simulink model "ModifiedBatteryModel3"  (R2019a)
settings: Solver=VariableStepAuto  StartTime=0.0  StopTime=10.0  RelTol=1e-3
libraries: fl_lib x6, nesl_utility x5
settings Model: Creator=nikos  LastModifiedBy=nikos

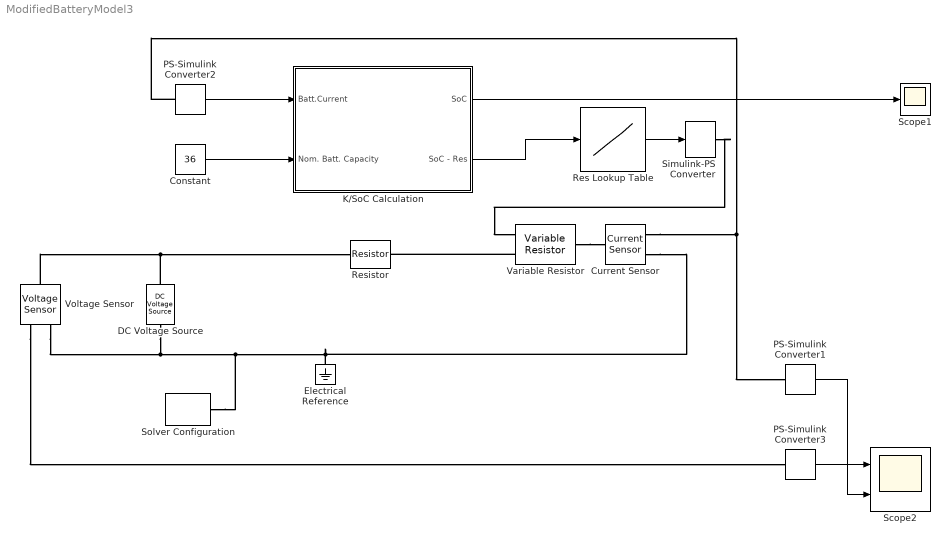
== system ModifiedBatteryModel3 ==
  Constant : Constant  Value=36
  Current Sensor : fl_lib/Electrical/Electrical Sensors/Current Sensor
  DC Voltage Source : fl_lib/Electrical/Electrical Sources/DC Voltage Source  v0=72 V
  Electrical Reference : fl_lib/Electrical/Electrical Elements/Electrical Reference
  K/SoC Calculation : Subsystem
  PS-Simulink Converter1 : nesl_utility/PS-Simulink Converter  PhysicalDomain=network_engine_domain  SubClassName=ps_output  LeftPortType=input  RightPortType=output  PseudoPeriodic=off  Frequencies=[]  Unit=1  AffineConversion=off
  PS-Simulink Converter2 : nesl_utility/PS-Simulink Converter  PhysicalDomain=network_engine_domain  SubClassName=ps_output  LeftPortType=input  RightPortType=output  PseudoPeriodic=off  Frequencies=[]  Unit=1  AffineConversion=off
  PS-Simulink Converter3 : nesl_utility/PS-Simulink Converter  PhysicalDomain=network_engine_domain  SubClassName=ps_output  LeftPortType=input  RightPortType=output  PseudoPeriodic=off  Frequencies=[]  Unit=1  AffineConversion=off
  Res Lookup Table : Lookup_n-D  NumberOfTableDimensions=1  BreakpointsForDimension1=[0, 10, 20, 30, 40, 50, 60, 70, 80, 90, 100]  Table=[0.011448, 0.011038, 0.011281, 0.011236, 0.010959, 0.010714, 0.010698, 0.010712, 0.010917, 0.011304, 0.011603]  InternalRulePriority=Speed  RndMeth=Simplest  InputSameDT=on
  Resistor : fl_lib/Electrical/Electrical Elements/Resistor  R=1.5 Ohm  i_specify=off  i_priority=High  i=0 A  i_nominal_specify=off  i_nominal_unit=A  i_nominal_value=1  v_specify=off  v_priority=High  v=0 V  v_nominal_specify=off  v_nominal_unit=V  v_nominal_value=1
  Scope1 : Scope
  Scope2 : Scope  NumInputPorts=2
  Simulink-PS Converter : nesl_utility/Simulink-PS Converter  PhysicalDomain=network_engine_domain  SubClassName=ps_input  LeftPortType=input  RightPortType=output  PseudoPeriodic=off  Frequencies=[]  NoiseDistribution=none  NoiseParameters=[]  Unit=1  AffineConversion=off  FilteringAndDerivatives=zero  SimscapeFilterOrder=1  InputFilterTimeConstant=0.001  UdotUserProvided=1
  Solver Configuration : nesl_utility/Solver Configuration  PhysicalDomain=network_engine_domain  SubClassName=solver  LeftPortType=input  RightPortType=generic  Tones=[]  Harmonics=[]  SimulateNoise=off  Profile=off  UseLocalSampling=off  EnableSwitchedLinearOptims=on  FrequencyDomain=off  UseCCode=off  RelTol=0.001  AbsTol=1e-06  MinStep=1e-09  ToWorkspace=off  RevertToSquareIcSolve=off  NumHomotopyIterations=100  PhasorMode=off  PhasorModeNumHarmonics=1  DoDC=off  ResidualTolerance=1e-09  UseLocalSolver=off  LocalSolverChoice=NE_BACKWARD_EULER_ADVANCER  LocalSolverSampleTime=0.001  DoFixedCost=off  MaxNonlinIter=3  MaxModeIter=2  LinearAlgebra=auto  EquationFormulation=NE_TIME_EF  DelaysMemoryBudget=1024  AutomaticFiltering=on  FilteringTimeConstant=0.001  PartitionStorageMethod=AS_NEEDED  PartitionMemoryBudget=1024  PartitionMethod=ROBUST
  Variable Resistor : fl_lib/Electrical/Electrical Elements/Variable Resistor  Rmin=0 Ohm  i_specify=off  i_priority=High  i=0 A  i_nominal_specify=off  i_nominal_unit=A  i_nominal_value=1  v_specify=off  v_priority=High  v=0 V  v_nominal_specify=off  v_nominal_unit=V  v_nominal_value=1
  Voltage Sensor : fl_lib/Electrical/Electrical Sensors/Voltage Sensor
  wires:
  Res Lookup Table/1 -> Simulink-PS Converter/1
  PS-Simulink Converter1/1 -> Scope2/2
  PS-Simulink Converter3/1 -> Scope2/1
  PS-Simulink Converter2/1 -> K/SoC Calculation/1(Batt.Current)
  Constant/1 -> K/SoC Calculation/2(Nom. Batt. Capacity)
  K/SoC Calculation/1(SoC) -> Scope1/1
  K/SoC Calculation/2(SoC - Res) -> Res Lookup Table/1
  connections:
  DC Voltage Source/LConn1 -- Voltage Sensor/LConn1 -- Resistor/LConn1
  DC Voltage Source/RConn1 -- Current Sensor/RConn2 -- Electrical Reference/LConn1 -- Solver Configuration/RConn1 -- Voltage Sensor/RConn2
  Variable Resistor/RConn1 -- Current Sensor/LConn1
  Simulink-PS Converter/RConn1 -- Variable Resistor/LConn1
  Variable Resistor/LConn2 -- Resistor/RConn1
  Voltage Sensor/RConn1 -- PS-Simulink Converter3/LConn1
  Current Sensor/RConn1 -- PS-Simulink Converter1/LConn1 -- PS-Simulink Converter2/LConn1

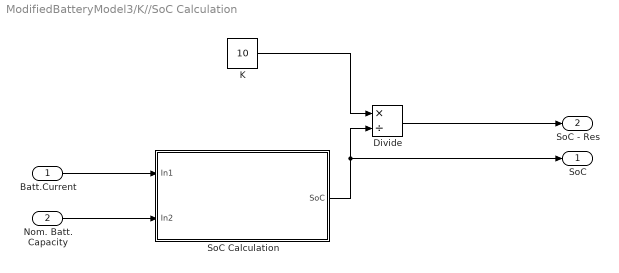
== system ModifiedBatteryModel3/K//SoC Calculation ==
  Batt.Current : Inport
  Nom. Batt. Capacity : Inport  Port=2
  Divide : Product  Inputs=*/
  K : Constant  Value=10
  SoC Calculation : Subsystem
  SoC : Outport
  SoC - Res : Outport  Port=2
  wires:
  SoC Calculation/1(" SoC") -> SoC/1, Divide/2
  Nom. Batt. Capacity/1 -> SoC Calculation/2(In2)
  K/1 -> Divide/1
  Divide/1 -> SoC - Res/1
  Batt.Current/1 -> SoC Calculation/1(In1)

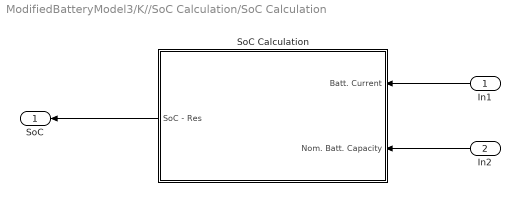
== system ModifiedBatteryModel3/K//SoC Calculation/SoC Calculation ==
  In1 : Inport
  In2 : Inport  Port=2
  SoC Calculation : Subsystem
  " SoC" : Outport
  wires:
  SoC Calculation/1(SoC - Res) -> " SoC"/1
  In1/1 -> SoC Calculation/1("Batt. Current ")
  In2/1 -> SoC Calculation/2("Nom. Batt. Capacity ")

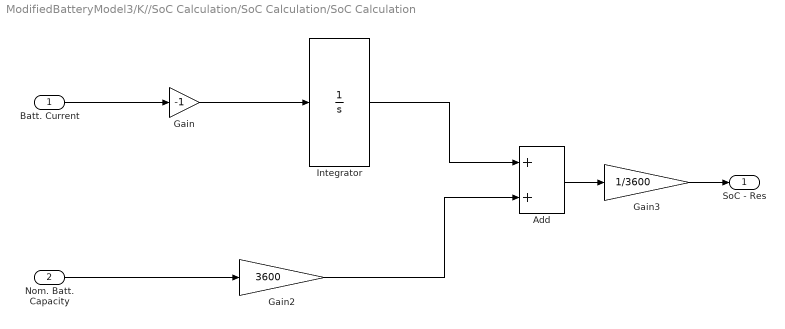
== system ModifiedBatteryModel3/K//SoC Calculation/SoC Calculation/SoC Calculation ==
  "Batt. Current " : Inport
  "Nom. Batt. Capacity " : Inport  Port=2  OutMin=0  OutMax=100
  Add : Sum
  Gain : Gain  Gain=-1
  Gain2 : Gain  Gain=3600
  Gain3 : Gain  Gain=1/3600
  Integrator : Integrator
  SoC - Res : Outport
  wires:
  Gain3/1 -> SoC - Res/1
  Integrator/1 -> Add/1
  Add/1 -> Gain3/1
  Gain2/1 -> Add/2
  "Nom. Batt. Capacity "/1 -> Gain2/1
  Gain/1 -> Integrator/1
  "Batt. Current "/1 -> Gain/1
